simulink model "Microstick_II_33EP128MC202_Drotek_I2C_MS5611_TempAndPressure"  (Simulink 7.5)
settings: Solver=FixedStepDiscrete  StartTime=0.0  StopTime=10.0  FixedStep=0.01  RelTol=1e-3
undefined symbols (not defined in the file or in its folder): A0, A4, B11, B8, B9, magnitude, Max, ms, P0, P15, P4, Pin, Resol, Slope1, Slope2, us
libraries: simulink x30, MCHP_Blockset x16
(part 2 of 2)

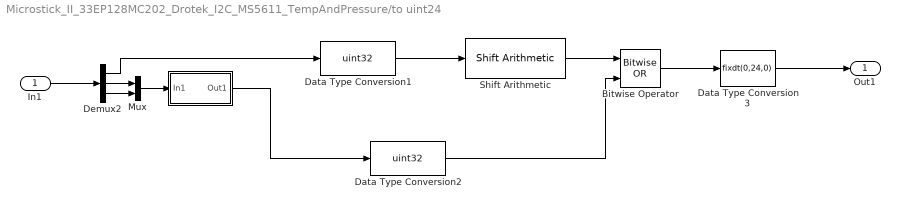
== system Microstick_II_33EP128MC202_Drotek_I2C_MS5611_TempAndPressure/to uint24 ==
  In1 : Inport
  " " : Subsystem
  Bitwise Operator : simulink/Logic and Bit Operations/Bitwise Operator  logicop=OR  UseBitMask=off  NumInputPorts=2  BitMask=bin2dec('11011001')  BitMaskRealWorld=Stored Integer
  Data Type Conversion1 : DataTypeConversion  OutDataTypeMode=uint32  OutDataTypeStr=uint32
  Data Type Conversion2 : DataTypeConversion  OutDataTypeMode=uint32  OutDataTypeStr=uint32
  Data Type Conversion3 : DataTypeConversion  OutDataTypeMode=Specify via dialog  OutDataType=fixdt(0,24,0)  OutDataTypeStr=fixdt(0,24,0)  ConvertRealWorld=Stored Integer (SI)
  Demux2 : Demux  Outputs=3
  Mux : Mux  Inputs=2
  Shift Arithmetic : simulink/Logic and Bit Operations/Shift Arithmetic  SystemSampleTime=-1  nBitShiftRight=-16  nBinPtShiftRight=0
  Out1 : Outport
  wires:
  In1/1 -> Demux2/1
  Shift Arithmetic/1 -> Bitwise Operator/1
  Demux2/1 -> Data Type Conversion1/1
  Mux/1 -> " "/1(In1)
  Demux2/2 -> Mux/1
  Bitwise Operator/1 -> Data Type Conversion3/1
  Demux2/3 -> Mux/2
  " "/1(Out1) -> Data Type Conversion2/1
  Data Type Conversion2/1 -> Bitwise Operator/2
  Data Type Conversion1/1 -> Shift Arithmetic/1
  Data Type Conversion3/1 -> Out1/1

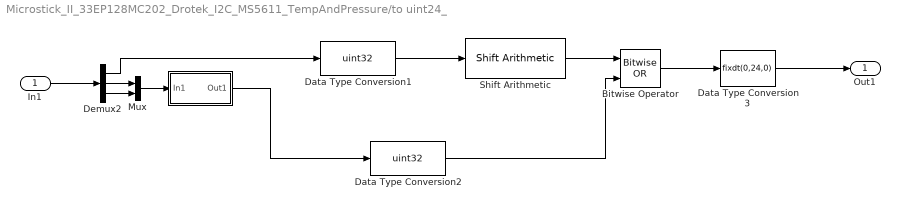
== system Microstick_II_33EP128MC202_Drotek_I2C_MS5611_TempAndPressure/to uint24_ ==
  In1 : Inport
  " " : Subsystem
  Bitwise Operator : simulink/Logic and Bit Operations/Bitwise Operator  logicop=OR  UseBitMask=off  NumInputPorts=2  BitMask=bin2dec('11011001')  BitMaskRealWorld=Stored Integer
  Data Type Conversion1 : DataTypeConversion  OutDataTypeMode=uint32  OutDataTypeStr=uint32
  Data Type Conversion2 : DataTypeConversion  OutDataTypeMode=uint32  OutDataTypeStr=uint32
  Data Type Conversion3 : DataTypeConversion  OutDataTypeMode=Specify via dialog  OutDataType=fixdt(0,24,0)  OutDataTypeStr=fixdt(0,24,0)  ConvertRealWorld=Stored Integer (SI)
  Demux2 : Demux  Outputs=3
  Mux : Mux  Inputs=2
  Shift Arithmetic : simulink/Logic and Bit Operations/Shift Arithmetic  SystemSampleTime=-1  nBitShiftRight=-16  nBinPtShiftRight=0
  Out1 : Outport
  wires:
  Data Type Conversion3/1 -> Out1/1
  Data Type Conversion1/1 -> Shift Arithmetic/1
  Data Type Conversion2/1 -> Bitwise Operator/2
  " "/1(Out1) -> Data Type Conversion2/1
  Demux2/3 -> Mux/2
  Bitwise Operator/1 -> Data Type Conversion3/1
  Demux2/2 -> Mux/1
  Mux/1 -> " "/1(In1)
  Demux2/1 -> Data Type Conversion1/1
  Shift Arithmetic/1 -> Bitwise Operator/1
  In1/1 -> Demux2/1

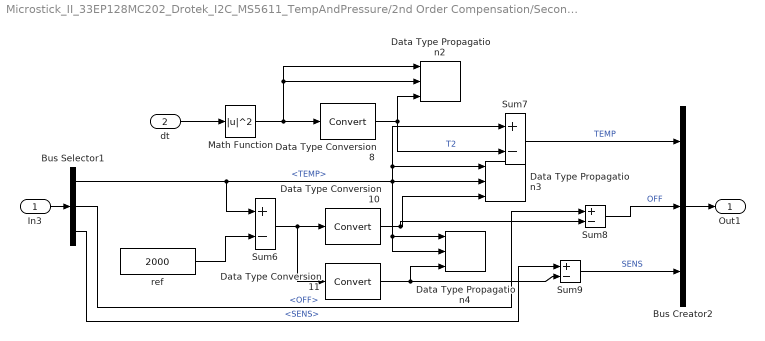
== system Microstick_II_33EP128MC202_Drotek_I2C_MS5611_TempAndPressure/2nd Order Compensation/Second Order Temp Compensation ==
  In3 : Inport
  dt : Inport  Port=2
  Bus Creator2 : BusCreator  Inputs=3
  Bus Selector1 : BusSelector  OutputSignals=TEMP,OFF,SENS
  Data Type Propagation2 : simulink/Signal Attributes/Data Type Propagation  PropDataType=fixdt(1, 16)  IfRefDouble=double  IfRefSingle=single  IsSigned=IsSigned1  NumBitsBase=NumBits1  NumBitsMult=1  NumBitsAdd=0  NumBitsAllowFinal=1:128  PropScaling=2^-10  ValuesUsedBestPrec=[5 -7]  SlopeBase=min([Slope1 Slope2])  SlopeMult=2^-31  SlopeAdd=0  BiasBase=Bias1  BiasMult=0  BiasAdd=0
  Data Type Propagation3 : simulink/Signal Attributes/Data Type Propagation  PropDataType=fixdt(1, 16)  IfRefDouble=double  IfRefSingle=single  IsSigned=IsSigned1  NumBitsBase=NumBits1  NumBitsMult=1  NumBitsAdd=0  NumBitsAllowFinal=1:128  PropScaling=2^-10  ValuesUsedBestPrec=[5 -7]  SlopeBase=Slope1  SlopeMult=5/2  SlopeAdd=0  BiasBase=Bias1  BiasMult=0  BiasAdd=0
  Data Type Propagation4 : simulink/Signal Attributes/Data Type Propagation  PropDataType=fixdt(1, 16)  IfRefDouble=double  IfRefSingle=single  IsSigned=IsSigned1  NumBitsBase=NumBits1  NumBitsMult=1  NumBitsAdd=0  NumBitsAllowFinal=1:128  PropScaling=2^-10  ValuesUsedBestPrec=[5 -7]  SlopeBase=Slope1  SlopeMult=5/4  SlopeAdd=0  BiasBase=Bias1  BiasMult=0  BiasAdd=0
  Data Type Conversion10 : DataTypeConversion  ConvertRealWorld=Stored Integer (SI)
  Data Type Conversion11 : DataTypeConversion  ConvertRealWorld=Stored Integer (SI)
  Data Type Conversion8 : DataTypeConversion  ConvertRealWorld=Stored Integer (SI)
  Math Function : Math  Operator=magnitude^2  OutDataTypeStr=Inherit: Inherit via back propagation  SaturateOnIntegerOverflow=on
  Sum{6..9} (4 alike) : Sum  Inputs=+-  OutDataTypeStr=Inherit: Same as accumulator
  ref : Constant  Value=2000  OutDataTypeMode=uint16  OutDataTypeStr=uint16
  Out1 : Outport
  wires:
  Bus Selector1/3 -> Sum9/1  "<SENS>"
  Sum8/1 -> Bus Creator2/2  "OFF"
  Bus Selector1/2 -> Sum8/1  "<OFF>"
  Sum7/1 -> Bus Creator2/1  "TEMP"
  Sum9/1 -> Bus Creator2/3  "SENS"
  Data Type Conversion11/1 -> Data Type Propagation4/3, Sum9/2
  ref/1 -> Sum6/2
  Bus Creator2/1 -> Out1/1
  Bus Selector1/1 -> Data Type Propagation3/1, Sum7/1, Data Type Propagation4/1, Data Type Propagation4/2, Data Type Propagation3/2, Sum6/1  "<TEMP>"
  Sum6/1 -> Data Type Conversion10/1, Data Type Conversion11/1
  In3/1 -> Bus Selector1/1
  Data Type Conversion8/1 -> Data Type Propagation2/3, Sum7/2  "T2"
  dt/1 -> Math Function/1
  Math Function/1 -> Data Type Conversion8/1, Data Type Propagation2/1, Data Type Propagation2/2
  Data Type Conversion10/1 -> Data Type Propagation3/3, Sum8/2

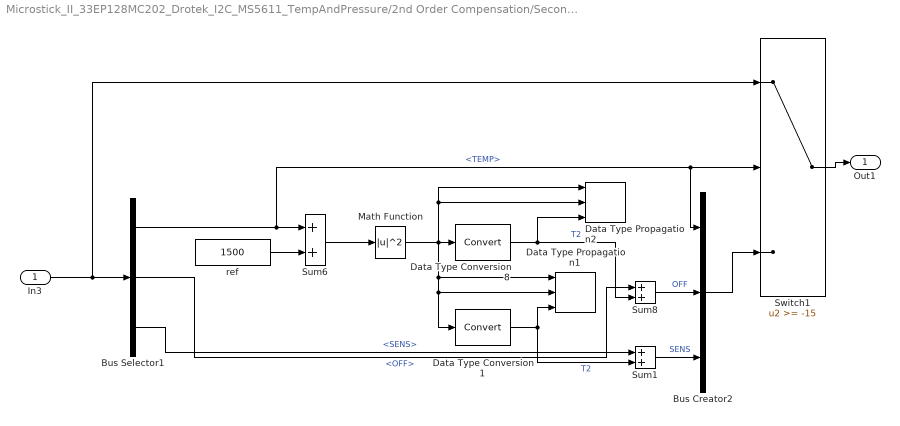
== system Microstick_II_33EP128MC202_Drotek_I2C_MS5611_TempAndPressure/2nd Order Compensation/Second Order Temp Compensation1 ==
  In3 : Inport
  Bus Creator2 : BusCreator  Inputs=3
  Bus Selector1 : BusSelector  OutputSignals=TEMP,OFF,SENS
  Data Type Propagation1 : simulink/Signal Attributes/Data Type Propagation  PropDataType=fixdt(1, 16)  IfRefDouble=double  IfRefSingle=single  IsSigned=IsSigned1  NumBitsBase=NumBits1  NumBitsMult=1  NumBitsAdd=0  NumBitsAllowFinal=1:128  PropScaling=2^-10  ValuesUsedBestPrec=[5 -7]  SlopeBase=min([Slope1 Slope2])  SlopeMult=11/2  SlopeAdd=0  BiasBase=Bias1  BiasMult=0  BiasAdd=0
  Data Type Propagation2 : simulink/Signal Attributes/Data Type Propagation  PropDataType=fixdt(1, 16)  IfRefDouble=double  IfRefSingle=single  IsSigned=IsSigned1  NumBitsBase=NumBits1  NumBitsMult=1  NumBitsAdd=0  NumBitsAllowFinal=1:128  PropScaling=2^-10  ValuesUsedBestPrec=[5 -7]  SlopeBase=min([Slope1 Slope2])  SlopeMult=7  SlopeAdd=0  BiasBase=Bias1  BiasMult=0  BiasAdd=0
  Data Type Conversion1 : DataTypeConversion  ConvertRealWorld=Stored Integer (SI)
  Data Type Conversion8 : DataTypeConversion  ConvertRealWorld=Stored Integer (SI)
  Math Function : Math  Operator=magnitude^2  OutDataTypeStr=Inherit: Inherit via back propagation  SaturateOnIntegerOverflow=on
  Sum1 : Sum  OutDataTypeStr=Inherit: Same as accumulator
  Sum6 : Sum  OutDataTypeStr=Inherit: Same as accumulator
  Sum8 : Sum  OutDataTypeStr=Inherit: Same as accumulator
  Switch1 : Switch  Threshold=-15  InputSameDT=on
  ref : Constant  Value=1500  OutDataTypeMode=uint16  OutDataTypeStr=uint16
  Out1 : Outport
  wires:
  In3/1 -> Switch1/1, Bus Selector1/1
  Sum8/1 -> Bus Creator2/2  "OFF"
  Bus Selector1/1 -> Switch1/2, Bus Creator2/1, Sum6/1  "<TEMP>"
  Math Function/1 -> Data Type Propagation1/1, Data Type Propagation1/2, Data Type Conversion1/1, Data Type Propagation2/2, Data Type Propagation2/1, Data Type Conversion8/1
  Data Type Conversion8/1 -> Sum8/2, Data Type Propagation2/3  "T2"
  Sum6/1 -> Math Function/1
  ref/1 -> Sum6/2
  Data Type Conversion1/1 -> Sum1/2, Data Type Propagation1/3  "T2"
  Sum1/1 -> Bus Creator2/3  "SENS"
  Bus Selector1/3 -> Sum1/1  "<SENS>"
  Bus Creator2/1 -> Switch1/3
  Switch1/1 -> Out1/1
  Bus Selector1/2 -> Sum8/1  "<OFF>"

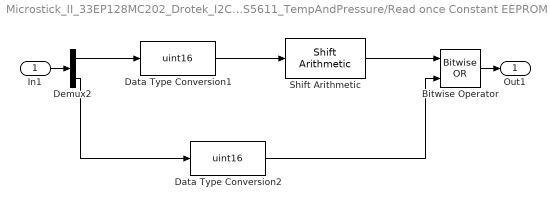
== system Microstick_II_33EP128MC202_Drotek_I2C_MS5611_TempAndPressure/Read once Constant EEPROM Calibration data From MS5611 (Blocking I2C blocks)/  ==
  In1 : Inport
  Bitwise Operator : simulink/Logic and Bit Operations/Bitwise Operator  logicop=OR  UseBitMask=off  NumInputPorts=2  BitMask=bin2dec('11011001')  BitMaskRealWorld=Stored Integer
  Data Type Conversion1 : DataTypeConversion  OutDataTypeMode=uint16  OutDataTypeStr=uint16
  Data Type Conversion2 : DataTypeConversion  OutDataTypeMode=uint16  OutDataTypeStr=uint16
  Demux2 : Demux  Outputs=2
  Shift Arithmetic : simulink/Logic and Bit Operations/Shift Arithmetic  SystemSampleTime=-1  nBitShiftRight=-8  nBinPtShiftRight=0
  Out1 : Outport
  wires:
  In1/1 -> Demux2/1
  Bitwise Operator/1 -> Out1/1
  Data Type Conversion1/1 -> Shift Arithmetic/1
  Demux2/2 -> Data Type Conversion2/1
  Shift Arithmetic/1 -> Bitwise Operator/1
  Demux2/1 -> Data Type Conversion1/1
  Data Type Conversion2/1 -> Bitwise Operator/2

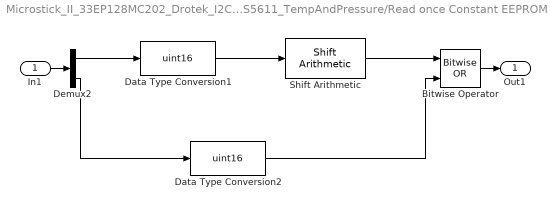
== system Microstick_II_33EP128MC202_Drotek_I2C_MS5611_TempAndPressure/Read once Constant EEPROM Calibration data From MS5611 (Blocking I2C blocks)/ 1 ==
  In1 : Inport
  Bitwise Operator : simulink/Logic and Bit Operations/Bitwise Operator  logicop=OR  UseBitMask=off  NumInputPorts=2  BitMask=bin2dec('11011001')  BitMaskRealWorld=Stored Integer
  Data Type Conversion1 : DataTypeConversion  OutDataTypeMode=uint16  OutDataTypeStr=uint16
  Data Type Conversion2 : DataTypeConversion  OutDataTypeMode=uint16  OutDataTypeStr=uint16
  Demux2 : Demux  Outputs=2
  Shift Arithmetic : simulink/Logic and Bit Operations/Shift Arithmetic  SystemSampleTime=-1  nBitShiftRight=-8  nBinPtShiftRight=0
  Out1 : Outport
  wires:
  Data Type Conversion2/1 -> Bitwise Operator/2
  Demux2/1 -> Data Type Conversion1/1
  Shift Arithmetic/1 -> Bitwise Operator/1
  Demux2/2 -> Data Type Conversion2/1
  Data Type Conversion1/1 -> Shift Arithmetic/1
  Bitwise Operator/1 -> Out1/1
  In1/1 -> Demux2/1

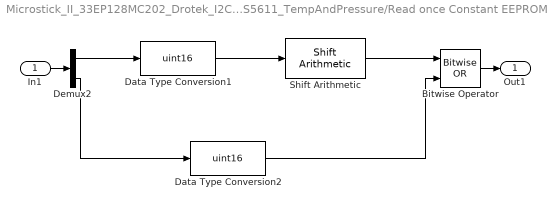
== system Microstick_II_33EP128MC202_Drotek_I2C_MS5611_TempAndPressure/Read once Constant EEPROM Calibration data From MS5611 (Blocking I2C blocks)/ 2 ==
  In1 : Inport
  Bitwise Operator : simulink/Logic and Bit Operations/Bitwise Operator  logicop=OR  UseBitMask=off  NumInputPorts=2  BitMask=bin2dec('11011001')  BitMaskRealWorld=Stored Integer
  Data Type Conversion1 : DataTypeConversion  OutDataTypeMode=uint16  OutDataTypeStr=uint16
  Data Type Conversion2 : DataTypeConversion  OutDataTypeMode=uint16  OutDataTypeStr=uint16
  Demux2 : Demux  Outputs=2
  Shift Arithmetic : simulink/Logic and Bit Operations/Shift Arithmetic  SystemSampleTime=-1  nBitShiftRight=-8  nBinPtShiftRight=0
  Out1 : Outport
  wires:
  In1/1 -> Demux2/1
  Bitwise Operator/1 -> Out1/1
  Data Type Conversion1/1 -> Shift Arithmetic/1
  Demux2/2 -> Data Type Conversion2/1
  Shift Arithmetic/1 -> Bitwise Operator/1
  Demux2/1 -> Data Type Conversion1/1
  Data Type Conversion2/1 -> Bitwise Operator/2

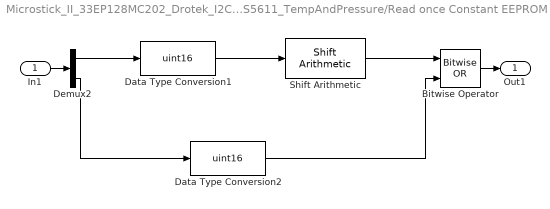
== system Microstick_II_33EP128MC202_Drotek_I2C_MS5611_TempAndPressure/Read once Constant EEPROM Calibration data From MS5611 (Blocking I2C blocks)/ 3 ==
  In1 : Inport
  Bitwise Operator : simulink/Logic and Bit Operations/Bitwise Operator  logicop=OR  UseBitMask=off  NumInputPorts=2  BitMask=bin2dec('11011001')  BitMaskRealWorld=Stored Integer
  Data Type Conversion1 : DataTypeConversion  OutDataTypeMode=uint16  OutDataTypeStr=uint16
  Data Type Conversion2 : DataTypeConversion  OutDataTypeMode=uint16  OutDataTypeStr=uint16
  Demux2 : Demux  Outputs=2
  Shift Arithmetic : simulink/Logic and Bit Operations/Shift Arithmetic  SystemSampleTime=-1  nBitShiftRight=-8  nBinPtShiftRight=0
  Out1 : Outport
  wires:
  Data Type Conversion2/1 -> Bitwise Operator/2
  Demux2/1 -> Data Type Conversion1/1
  Shift Arithmetic/1 -> Bitwise Operator/1
  Demux2/2 -> Data Type Conversion2/1
  Data Type Conversion1/1 -> Shift Arithmetic/1
  Bitwise Operator/1 -> Out1/1
  In1/1 -> Demux2/1

== system Microstick_II_33EP128MC202_Drotek_I2C_MS5611_TempAndPressure/Read once Constant EEPROM Calibration data From MS5611 (Blocking I2C blocks)/ 4 ==
  In1 : Inport
  Bitwise Operator : simulink/Logic and Bit Operations/Bitwise Operator  logicop=OR  UseBitMask=off  NumInputPorts=2  BitMask=bin2dec('11011001')  BitMaskRealWorld=Stored Integer
  Data Type Conversion1 : DataTypeConversion  OutDataTypeMode=uint16  OutDataTypeStr=uint16
  Data Type Conversion2 : DataTypeConversion  OutDataTypeMode=uint16  OutDataTypeStr=uint16
  Demux2 : Demux  Outputs=2
  Shift Arithmetic : simulink/Logic and Bit Operations/Shift Arithmetic  SystemSampleTime=-1  nBitShiftRight=-8  nBinPtShiftRight=0
  Out1 : Outport
  wires:
  In1/1 -> Demux2/1
  Bitwise Operator/1 -> Out1/1
  Data Type Conversion1/1 -> Shift Arithmetic/1
  Demux2/2 -> Data Type Conversion2/1
  Shift Arithmetic/1 -> Bitwise Operator/1
  Demux2/1 -> Data Type Conversion1/1
  Data Type Conversion2/1 -> Bitwise Operator/2

== system Microstick_II_33EP128MC202_Drotek_I2C_MS5611_TempAndPressure/Read once Constant EEPROM Calibration data From MS5611 (Blocking I2C blocks)/ 5 ==
  In1 : Inport
  Bitwise Operator : simulink/Logic and Bit Operations/Bitwise Operator  logicop=OR  UseBitMask=off  NumInputPorts=2  BitMask=bin2dec('11011001')  BitMaskRealWorld=Stored Integer
  Data Type Conversion1 : DataTypeConversion  OutDataTypeMode=uint16  OutDataTypeStr=uint16
  Data Type Conversion2 : DataTypeConversion  OutDataTypeMode=uint16  OutDataTypeStr=uint16
  Demux2 : Demux  Outputs=2
  Shift Arithmetic : simulink/Logic and Bit Operations/Shift Arithmetic  SystemSampleTime=-1  nBitShiftRight=-8  nBinPtShiftRight=0
  Out1 : Outport
  wires:
  Data Type Conversion2/1 -> Bitwise Operator/2
  Demux2/1 -> Data Type Conversion1/1
  Shift Arithmetic/1 -> Bitwise Operator/1
  Demux2/2 -> Data Type Conversion2/1
  Data Type Conversion1/1 -> Shift Arithmetic/1
  Bitwise Operator/1 -> Out1/1
  In1/1 -> Demux2/1

== system Microstick_II_33EP128MC202_Drotek_I2C_MS5611_TempAndPressure/to uint24/  ==
  In1 : Inport
  Bitwise Operator : simulink/Logic and Bit Operations/Bitwise Operator  logicop=OR  UseBitMask=off  NumInputPorts=2  BitMask=bin2dec('11011001')  BitMaskRealWorld=Stored Integer
  Data Type Conversion1 : DataTypeConversion  OutDataTypeMode=uint16  OutDataTypeStr=uint16
  Data Type Conversion2 : DataTypeConversion  OutDataTypeMode=uint16  OutDataTypeStr=uint16
  Demux2 : Demux  Outputs=2
  Shift Arithmetic : simulink/Logic and Bit Operations/Shift Arithmetic  SystemSampleTime=-1  nBitShiftRight=-8  nBinPtShiftRight=0
  Out1 : Outport
  wires:
  Data Type Conversion2/1 -> Bitwise Operator/2
  Demux2/1 -> Data Type Conversion1/1
  Shift Arithmetic/1 -> Bitwise Operator/1
  Demux2/2 -> Data Type Conversion2/1
  Data Type Conversion1/1 -> Shift Arithmetic/1
  Bitwise Operator/1 -> Out1/1
  In1/1 -> Demux2/1

== system Microstick_II_33EP128MC202_Drotek_I2C_MS5611_TempAndPressure/to uint24_/  ==
  In1 : Inport
  Bitwise Operator : simulink/Logic and Bit Operations/Bitwise Operator  logicop=OR  UseBitMask=off  NumInputPorts=2  BitMask=bin2dec('11011001')  BitMaskRealWorld=Stored Integer
  Data Type Conversion1 : DataTypeConversion  OutDataTypeMode=uint16  OutDataTypeStr=uint16
  Data Type Conversion2 : DataTypeConversion  OutDataTypeMode=uint16  OutDataTypeStr=uint16
  Demux2 : Demux  Outputs=2
  Shift Arithmetic : simulink/Logic and Bit Operations/Shift Arithmetic  SystemSampleTime=-1  nBitShiftRight=-8  nBinPtShiftRight=0
  Out1 : Outport
  wires:
  In1/1 -> Demux2/1
  Bitwise Operator/1 -> Out1/1
  Data Type Conversion1/1 -> Shift Arithmetic/1
  Demux2/2 -> Data Type Conversion2/1
  Shift Arithmetic/1 -> Bitwise Operator/1
  Demux2/1 -> Data Type Conversion1/1
  Data Type Conversion2/1 -> Bitwise Operator/2
